simulink library "INT_AirCtl_Mon"  (R2016b)
settings: Solver=VariableStepAuto  StartTime=0.0  StopTime=10.0  RelTol=1e-3
settings Model: Creator=guanxiaoxing  LastModifiedBy=guanxiaoxing

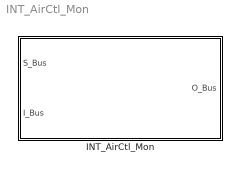
== system INT_AirCtl_Mon ==
  INT_AirCtl_Mon : Subsystem

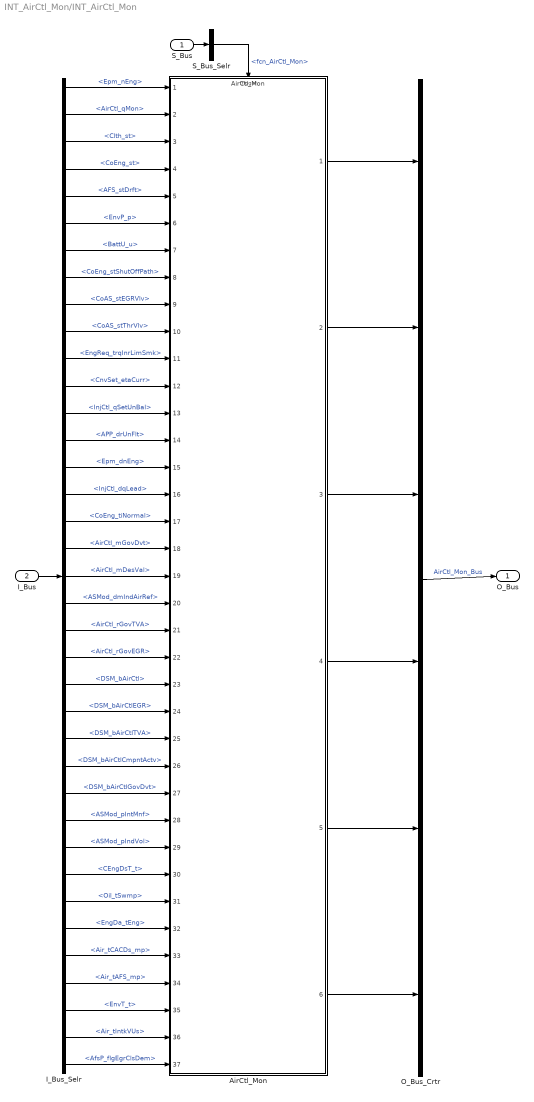
== system INT_AirCtl_Mon/INT_AirCtl_Mon ==
  S_Bus : Inport
  I_Bus : Inport  Port=2
  AirCtl_Mon : ModelReference  ModelNameDialog=AirCtl_Mon  SimulationMode=Normal  ModelReferenceVersion=1.92  TriggerPortName=function  TriggerPortTriggerType=function-call  TriggerPortStatesWhenEnabling=held
  I_Bus_Selr : BusSelector  OutputSignals=Epm_nEng,AirCtl_qMon,Clth_st,CoEng_st,AFS_stDrft,EnvP_p,BattU_u,CoEng_stShutOffPath,CoAS_stEGRVlv,CoAS_stThrVlv,EngReq_trqInrLimSmk,CnvSet_etaCurr,InjCtl_qSetUnBal,APP_drUnFlt,Epm_dnEng,InjCtl_dqLead,CoEng_tiNormal,AirCtl_mGovDvt,AirCtl_mDesVal,ASMod_dmIndAirRef,AirCtl_rGovTVA,AirCtl_rGovEGR,DSM_bAirCtl,DSM_bAirCtlEGR,DSM_bAirCtlTVA,DSM_bAirCtlCmpntActv,DSM_bAirCtlGovDvt,ASMod_pIntMnf,ASMod_pIndVol,CEngDsT_t,Oil_tSwmp,EngDa_tEng,Air_tCACDs_mp,Air_tAFS_mp,EnvT_t,Air_tIntkVUs,AfsP_flgEgrClsDem
  O_Bus_Crtr : BusCreator  Inputs=6
  S_Bus_Selr : BusSelector  OutputSignals=fcn_AirCtl_Mon
  O_Bus : Outport
  wires:
  S_Bus_Selr/1 -> AirCtl_Mon/Trigger  "<fcn_AirCtl_Mon>"
  S_Bus/1 -> S_Bus_Selr/1
  I_Bus/1 -> I_Bus_Selr/1
  I_Bus_Selr/1 -> AirCtl_Mon/1  "<Epm_nEng>"
  I_Bus_Selr/2 -> AirCtl_Mon/2  "<AirCtl_qMon>"
  I_Bus_Selr/3 -> AirCtl_Mon/3  "<Clth_st>"
  I_Bus_Selr/4 -> AirCtl_Mon/4  "<CoEng_st>"
  I_Bus_Selr/5 -> AirCtl_Mon/5  "<AFS_stDrft>"
  I_Bus_Selr/6 -> AirCtl_Mon/6  "<EnvP_p>"
  I_Bus_Selr/7 -> AirCtl_Mon/7  "<BattU_u>"
  I_Bus_Selr/8 -> AirCtl_Mon/8  "<CoEng_stShutOffPath>"
  I_Bus_Selr/9 -> AirCtl_Mon/9  "<CoAS_stEGRVlv>"
  I_Bus_Selr/10 -> AirCtl_Mon/10  "<CoAS_stThrVlv>"
  I_Bus_Selr/11 -> AirCtl_Mon/11  "<EngReq_trqInrLimSmk>"
  I_Bus_Selr/12 -> AirCtl_Mon/12  "<CnvSet_etaCurr>"
  I_Bus_Selr/13 -> AirCtl_Mon/13  "<InjCtl_qSetUnBal>"
  I_Bus_Selr/14 -> AirCtl_Mon/14  "<APP_drUnFlt>"
  I_Bus_Selr/15 -> AirCtl_Mon/15  "<Epm_dnEng>"
  I_Bus_Selr/16 -> AirCtl_Mon/16  "<InjCtl_dqLead>"
  I_Bus_Selr/17 -> AirCtl_Mon/17  "<CoEng_tiNormal>"
  I_Bus_Selr/18 -> AirCtl_Mon/18  "<AirCtl_mGovDvt>"
  I_Bus_Selr/19 -> AirCtl_Mon/19  "<AirCtl_mDesVal>"
  I_Bus_Selr/20 -> AirCtl_Mon/20  "<ASMod_dmIndAirRef>"
  I_Bus_Selr/21 -> AirCtl_Mon/21  "<AirCtl_rGovTVA>"
  I_Bus_Selr/22 -> AirCtl_Mon/22  "<AirCtl_rGovEGR>"
  I_Bus_Selr/23 -> AirCtl_Mon/23  "<DSM_bAirCtl>"
  I_Bus_Selr/24 -> AirCtl_Mon/24  "<DSM_bAirCtlEGR>"
  I_Bus_Selr/25 -> AirCtl_Mon/25  "<DSM_bAirCtlTVA>"
  I_Bus_Selr/26 -> AirCtl_Mon/26  "<DSM_bAirCtlCmpntActv>"
  I_Bus_Selr/27 -> AirCtl_Mon/27  "<DSM_bAirCtlGovDvt>"
  I_Bus_Selr/28 -> AirCtl_Mon/28  "<ASMod_pIntMnf>"
  I_Bus_Selr/29 -> AirCtl_Mon/29  "<ASMod_pIndVol>"
  I_Bus_Selr/30 -> AirCtl_Mon/30  "<CEngDsT_t>"
  I_Bus_Selr/31 -> AirCtl_Mon/31  "<Oil_tSwmp>"
  I_Bus_Selr/32 -> AirCtl_Mon/32  "<EngDa_tEng>"
  I_Bus_Selr/33 -> AirCtl_Mon/33  "<Air_tCACDs_mp>"
  I_Bus_Selr/34 -> AirCtl_Mon/34  "<Air_tAFS_mp>"
  I_Bus_Selr/35 -> AirCtl_Mon/35  "<EnvT_t>"
  I_Bus_Selr/36 -> AirCtl_Mon/36  "<Air_tIntkVUs>"
  I_Bus_Selr/37 -> AirCtl_Mon/37  "<AfsP_flgEgrClsDem>"
  O_Bus_Crtr/1 -> O_Bus/1  "AirCtl_Mon_Bus"
  AirCtl_Mon/1 -> O_Bus_Crtr/1
  AirCtl_Mon/2 -> O_Bus_Crtr/2
  AirCtl_Mon/3 -> O_Bus_Crtr/3
  AirCtl_Mon/4 -> O_Bus_Crtr/4
  AirCtl_Mon/5 -> O_Bus_Crtr/5
  AirCtl_Mon/6 -> O_Bus_Crtr/6
